simulink model "Questao1_2"  (R2023b)
settings: Solver=VariableStepAuto  StartTime=0.0  StopTime=0.1  RelTol=1e-3
undefined symbols (not defined in the file): b, f_final, f_inicial, fa, k, m, mi, t_inicial
settings Model: Creator=klaus
settings SolverCC: AlgebraicLoopSolver=TrustRegion
settings DebuggingCC: UnconnectedInputMsg=warning  UnconnectedOutputMsg=warning  UnconnectedLineMsg=warning
settings ModelReferenceCC: EnableRefExpFcnMdlSchedulingChecks=on

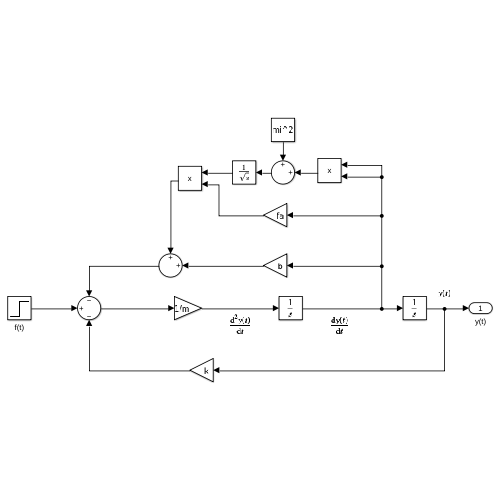
[thumbnail: Simulink's stored preview of the top-level diagram]
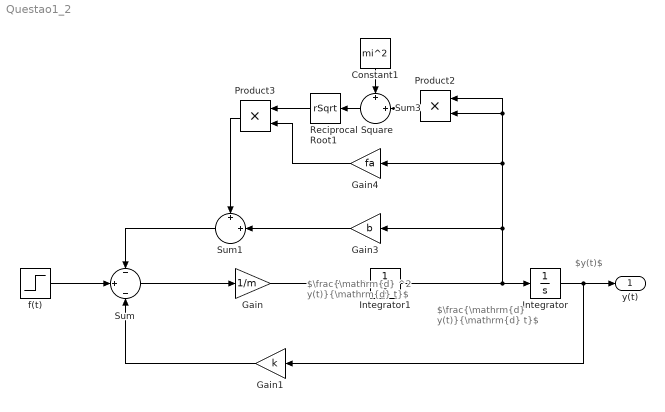
== system Questao1_2 ==
  note: $y(t)$
  note: $\frac{\mathrm{d} y(t)}{\mathrm{d} t}$
  note: $\frac{\mathrm{d} ^2 y(t)}{\mathrm{d} t}$
  Constant1 : Constant  Value=mi^2
  Gain : Gain  Gain=1/m
  Gain1 : Gain  Gain=k
  Gain3 : Gain  Gain=b
  Gain4 : Gain  Gain=fa
  Integrator : Integrator
  Integrator1 : Integrator
  Product2 : Product
  Product3 : Product
  Reciprocal Square Root1 : Sqrt  Operator=rSqrt
  Sum : Sum  Inputs=-|+|-
  Sum1 : Sum  Inputs=+|+||
  Sum3 : Sum  Inputs=+|+||
  f(t) : Step  Time=t_inicial  Before=f_inicial  After=f_final  SampleTime=0
  y(t) : Outport
  wires:
  f(t)/1 -> Sum/2
  Sum/1 -> Gain/1
  Gain/1 -> Integrator1/1
  Integrator1/1 -> Integrator/1, Gain3/1, Gain4/1, Product2/2, Product2/1
  Integrator/1 -> Gain1/1, y(t)/1
  Gain1/1 -> Sum/3
  Gain3/1 -> Sum1/2
  Sum1/1 -> Sum/1
  Product2/1 -> Sum3/2
  Constant1/1 -> Sum3/1
  Sum3/1 -> Reciprocal Square Root1/1
  Reciprocal Square Root1/1 -> Product3/1
  Gain4/1 -> Product3/2
  Product3/1 -> Sum1/1
